simulink model "Subsystem"  (R2020a)
settings: Solver=FixedStepAuto  StartTime=0.0  StopTime=10.0  FixedStep=0.2  RelTol=1e-3
model workspace (MAT data in the model file):
  Gain_A = 2
  Gain_B = -3
  Gain_C = -4
  Gain_D = 5
settings Model: Creator=INDRAJIT MARATHE  LastModifiedBy=INDRAJIT MARATHE
settings DataIOCC: SaveOutput=off  SaveTime=off

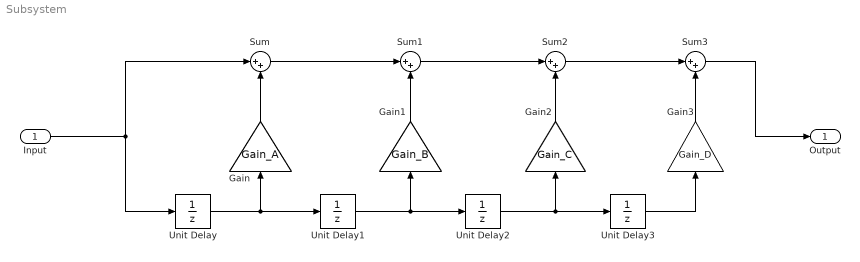
== system Subsystem ==
  Input : Inport  OutDataTypeStr=double  PortDimensions=1  SampleTime=[0.20000000000000001,0]
  Gain : Gain  Gain=Gain_A
  Gain1 : Gain  Gain=Gain_B
  Gain2 : Gain  Gain=Gain_C
  Gain3 : Gain  Gain=Gain_D
  Sum{,1..3} (4 alike) : Sum  Inputs=|++
  Unit Delay{,1..3} (4 alike) : UnitDelay  SampleTime=-1  HasFrameUpgradeWarning=on
  Output : Outport  OutDataTypeStr=double  PortDimensions=1  SampleTime=[0.20000000000000001,0]
  wires:
  Sum3/1 -> Output/1
  Unit Delay3/1 -> Gain3/1
  Gain/1 -> Sum/2
  Input/1 -> Unit Delay/1, Sum/1
  Unit Delay1/1 -> Unit Delay2/1, Gain1/1
  Sum/1 -> Sum1/1
  Sum1/1 -> Sum2/1
  Gain1/1 -> Sum1/2
  Gain2/1 -> Sum2/2
  Gain3/1 -> Sum3/2
  Unit Delay2/1 -> Unit Delay3/1, Gain2/1
  Unit Delay/1 -> Unit Delay1/1, Gain/1
  Sum2/1 -> Sum3/1
